simulink model "CDPM"  (R2013a)
settings: Solver=ode45  StartTime=0.0  StopTime=30  RelTol=1e-3
undefined symbols (not defined in the file): A
libraries: fl_lib x52, dspmtrx3 x21, nesl_utility x16, vrlib x12, simulink x9, elec_lib x8, sdl_lib x4, dspsigops x4, elec_controlled_stepper_lib x4
(part 2 of 2)

== system CDPM/NM4Y /Subsystem/Meas 1 ==
  Electrical Reference : fl_lib/Electrical/Electrical Elements/Electrical Reference  i_Log=off  LocalVarNames=|i  LocalVarDescs=|i  LocalVarLogging=[]
  PS-Simulink Converter : nesl_utility/PS-Simulink Converter  PhysicalDomain=network_engine_domain  SubClassName=ps_output  LeftPortType=input  RightPortType=output  PseudoPeriodic=off  Frequencies=[]  Unit=V  AffineConversion=off
  Voltage Sensor : fl_lib/Electrical/Electrical Sensors/Voltage Sensor  i1_Log=off  v1_Log=off  LocalVarNames=|i1|v1  LocalVarDescs=|i1|v1  LocalVarLogging=[]
  V : PMIOPort  Port=1  Side=Left
  SL : Outport
  wires:
  PS-Simulink Converter/1 -> SL/1
  connections:
  V/RConn1 -- Voltage Sensor/LConn1
  Electrical Reference/LConn1 -- Voltage Sensor/RConn2
  Voltage Sensor/RConn1 -- PS-Simulink Converter/LConn1

== system CDPM/NM4Y /Subsystem/Meas 2 ==
  Electrical Reference : fl_lib/Electrical/Electrical Elements/Electrical Reference  i_Log=off  LocalVarNames=|i  LocalVarDescs=|i  LocalVarLogging=[]
  PS-Simulink Converter : nesl_utility/PS-Simulink Converter  PhysicalDomain=network_engine_domain  SubClassName=ps_output  LeftPortType=input  RightPortType=output  PseudoPeriodic=off  Frequencies=[]  Unit=V  AffineConversion=off
  Voltage Sensor : fl_lib/Electrical/Electrical Sensors/Voltage Sensor  i1_Log=off  v1_Log=off  LocalVarNames=|i1|v1  LocalVarDescs=|i1|v1  LocalVarLogging=[]
  V : PMIOPort  Port=1  Side=Left
  SL : Outport
  wires:
  PS-Simulink Converter/1 -> SL/1
  connections:
  V/RConn1 -- Voltage Sensor/LConn1
  Electrical Reference/LConn1 -- Voltage Sensor/RConn2
  Voltage Sensor/RConn1 -- PS-Simulink Converter/LConn1

== system CDPM/NM4Y /Subsystem/Stepper Controller ==
  Ref : Inport
  Position Controller : elec_controlled_stepper_lib/Position Controller
  PWM : PMIOPort  Port=1  Side=Right
  0v : PMIOPort  Port=2  Side=Right
  REV : PMIOPort  Port=3  Side=Right
  wires:
  Ref/1 -> Position Controller/1
  connections:
  Position Controller/RConn1 -- PWM/RConn1
  Position Controller/RConn2 -- 0v/RConn1
  Position Controller/RConn3 -- REV/RConn1

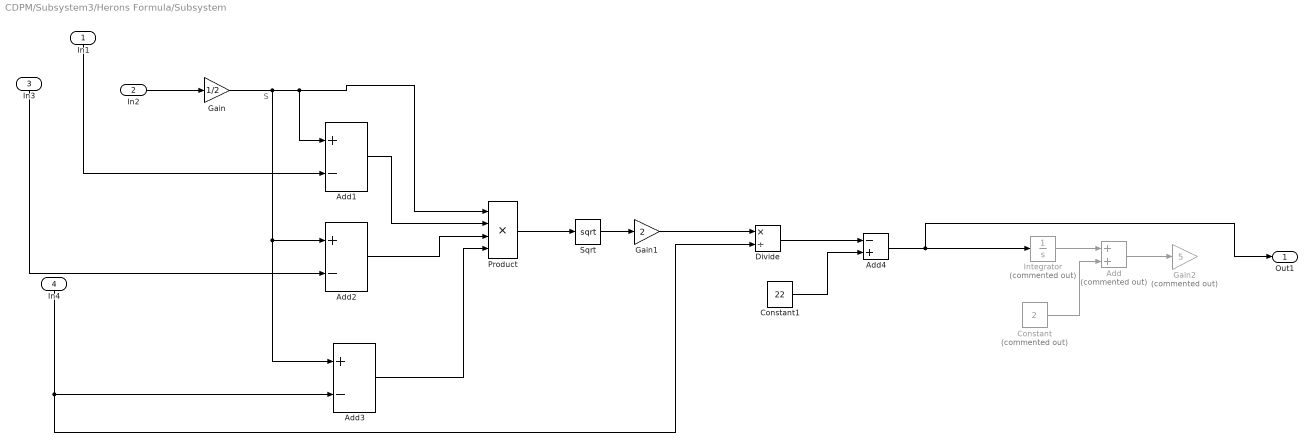
== system CDPM/Subsystem3/Herons Formula/Subsystem ==
  note: S
  In1 : Inport
  In2 : Inport  Port=2
  In3 : Inport  Port=3
  In4 : Inport  Port=4
  Add : Sum  Commented=on
  Add1 : Sum  Inputs=+-
  Add2 : Sum  Inputs=+-
  Add3 : Sum  Inputs=+-
  Add4 : Sum  Inputs=-+
  Constant : Constant  Commented=on  Value=2
  Constant1 : Constant  Value=22
  Divide : Product  Inputs=*/
  Gain : Gain  Gain=1/2
  Gain1 : Gain  Gain=2
  Gain2 : Gain  Commented=on  Gain=5
  Integrator : Integrator  Commented=on
  Product : Product  Inputs=4
  Sqrt : Sqrt  SaturateOnIntegerOverflow=on
  Out1 : Outport
  wires:
  Gain1/1 -> Divide/1
  In2/1 -> Gain/1
  Gain/1 -> Add3/1, Add2/1, Add1/1, Product/1
  Sqrt/1 -> Gain1/1
  Add1/1 -> Product/2
  Add2/1 -> Product/3
  Constant1/1 -> Add4/2
  Add3/1 -> Product/4
  Product/1 -> Sqrt/1
  Divide/1 -> Add4/1
  In1/1 -> Add1/2
  In4/1 -> Divide/2, Add3/2
  In3/1 -> Add2/2
  Add4/1 -> Out1/1, Integrator/1
  Integrator/1 -> Add/1
  Constant/1 -> Add/2
  Add/1 -> Gain2/1

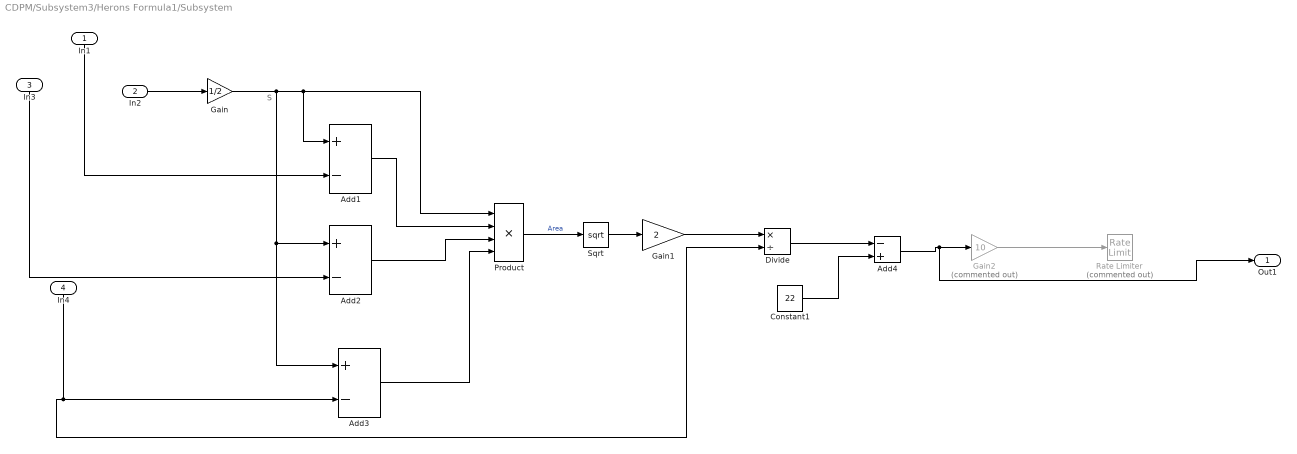
== system CDPM/Subsystem3/Herons Formula1/Subsystem ==
  note: S
  In1 : Inport
  In2 : Inport  Port=2
  In3 : Inport  Port=3
  In4 : Inport  Port=4
  Add1 : Sum  Inputs=+-
  Add2 : Sum  Inputs=+-
  Add3 : Sum  Inputs=+-
  Add4 : Sum  Inputs=-+
  Constant1 : Constant  Value=22
  Divide : Product  Inputs=*/
  Gain : Gain  Gain=1/2
  Gain1 : Gain  Gain=2
  Gain2 : Gain  Commented=on  Gain=10
  Product : Product  Inputs=4
  Rate Limiter : RateLimiter  Commented=on  RisingSlewLimit=50  FallingSlewLimit=-50  SampleTimeMode=inherited
  Sqrt : Sqrt  SaturateOnIntegerOverflow=on
  Out1 : Outport
  wires:
  Gain1/1 -> Divide/1
  In2/1 -> Gain/1
  Gain/1 -> Add3/1, Add2/1, Add1/1, Product/1
  Sqrt/1 -> Gain1/1
  Add1/1 -> Product/2
  Add2/1 -> Product/3
  Constant1/1 -> Add4/2
  Add3/1 -> Product/4
  Product/1 -> Sqrt/1  "Area"
  Divide/1 -> Add4/1
  In1/1 -> Add1/2
  In4/1 -> Divide/2, Add3/2
  In3/1 -> Add2/2
  Add4/1 -> Out1/1, Gain2/1
  Gain2/1 -> Rate Limiter/1

== matlab function CDPM/Main Control /Main Function  ==
  data: u input; i input; Cpos input; cout output; Dpos output; y output; x output
function [cout,Dpos,y,x] = fcn(u,i,Cpos)
%#codegen
limit=20;
npos=[0 0 0 0];
Dpos=[0 0 0 0];
    x=u(1,i);
    y=u(2,i);
    npos(1)=sqrt((x+limit).^2+(y-limit).^2);
    npos(2)=sqrt((x-limit).^2+(y-limit).^2);
    npos(3)=sqrt((x+limit).^2+(y+limit).^2);
	npos(4)=sqrt((x-limit).^2+(y+limit).^2);
    Dpos=Cpos-npos;
    cout=npos;

== matlab function CDPM/Main Control /Test Case Generator  ==
  data: y output; Cpos output
function [y,Cpos]= fcn
%#codegen
p=[-15 -5 5 15];
p1=horzcat(p,p);
p2=horzcat(p1,p1);
z=[15 15 15 15];
t=[5 5 5 5];
z1=horzcat(z,t);
t=-t;
z2=horzcat(z1,t);
t=t+10;
t=t-20;
z3=horzcat(z2,t);
z4=vertcat(p2,z3);
y = z4;
Cpos=[30,30,30,30]
end
